simulink model "ClosedLoop_ssPlant_Kcont"  (R2017a)
settings: Solver=VariableStepAuto  StartTime=0.0  StopTime=10.0  RelTol=1e-3
settings Model: Creator=manzand  LastModifiedBy=manzand

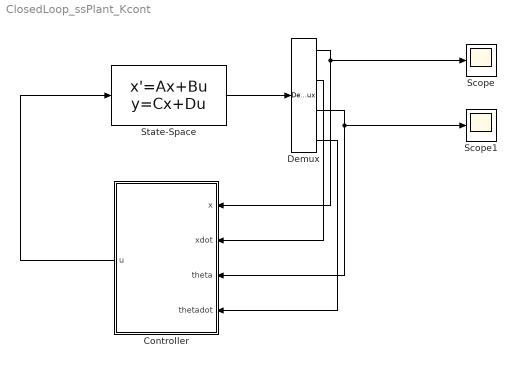
== system ClosedLoop_ssPlant_Kcont ==
  Controller : Subsystem
  Demux : Demux
  Scope : Scope
  Scope1 : Scope
  State-Space : StateSpace  A="[10.277464798470250  0.593654749979796  0.003358104029173  1.64532577728261e-14;  -14.6117489467771  -4.73043929988204  -0.0675348684607735  1.43619477870884e-14;  -0.0756273760098102  -0.220528039127163  -0.613790641123685  -6.20168844754436e-16; 0 0 0 -100]"  B=|  C="[-0.340562613667800  -0.435153403386864  -13.5706224450963  -3.38051638789472e-16; -5.85037462905811  0.581501260152669  0.428559339277117  2.04159142198002e-15;  0.554980878334768 -1.17895207022420  0.238359805913809  3.16762570985349e-17;  5.35950097269269  3.85737621442000  3.65943497063795  -5.66486175322742e-15]"  D=|  X0=0
      B=|
      | [-0.305503949564489
      | ;-0.408442923486334;
      | 0.00160131928946421;
      | 3.53641652353394e-17]
      D=|
      | [-0.00212878534341077;
      | -0.0142874533085508;
      | -0.00259724752489116;
      | 0.0283972893578094]
  wires:
  State-Space/1 -> Demux/1
  Demux/1 -> Scope/1, Controller/1(x)
  Demux/2 -> Controller/2(xdot)
  Demux/3 -> Scope1/1, Controller/3(theta)
  Demux/4 -> Controller/4(thetadot)
  Controller/1(u) -> State-Space/1

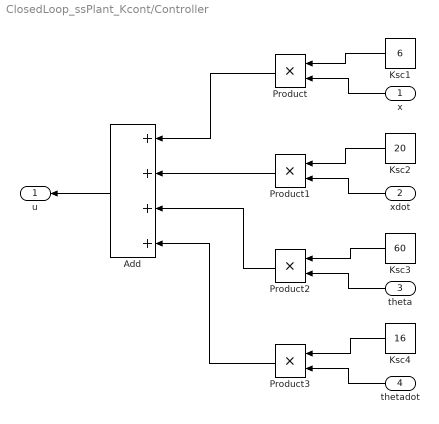
== system ClosedLoop_ssPlant_Kcont/Controller ==
  x : Inport
  xdot : Inport  Port=2
  theta : Inport  Port=3
  thetadot : Inport  Port=4
  Add : Sum  Inputs=++++
  Ksc1 : Constant  Value=6
  Ksc2 : Constant  Value=20
  Ksc3 : Constant  Value=60
  Ksc4 : Constant  Value=16
  Product{,1..3} (4 alike) : Product
  u : Outport
  wires:
  theta/1 -> Product2/2
  Ksc4/1 -> Product3/1
  Ksc1/1 -> Product/1
  xdot/1 -> Product1/2
  Ksc2/1 -> Product1/1
  x/1 -> Product/2
  thetadot/1 -> Product3/2
  Ksc3/1 -> Product2/1
  Product/1 -> Add/1
  Product3/1 -> Add/4
  Product2/1 -> Add/3
  Add/1 -> u/1
  Product1/1 -> Add/2
